simulink model "RLmodel"  (R2025b)
settings: Solver=FixedStepAuto  StartTime=0.0  StopTime=20.05  FixedStep=0.001  RelTol=1e-5  AbsTol=1e-6
model workspace (MAT data in the model file):
  I = 0
  c = 0
  g = 9.81
  l = 1
  m = 1
  max_tau = 2
undefined symbols (not defined in the file): x0
settings Model: Creator=The MathWorks, Inc.  LastModifiedBy=lengj
settings SolverCC: AutoScaleAbsTol=off  AlgebraicLoopSolver=TrustRegion
settings DataIOCC: LimitDataPoints=on  SaveFormat=Array  SaveState=on
settings OptimizationCC: BlockReduction=off  BooleanDataType=off  LifeSpan=inf
settings DebuggingCC: SaveWithParameterizedLinksMsg=none  SignalResolutionControl=TryResolveAllWithWarning  UnconnectedInputMsg=warning  UnconnectedOutputMsg=warning  UnconnectedLineMsg=warning  SFUnexpectedBacktrackingDiag=warning  SFNoUnconditionalDefaultTransitionDiag=warning  SFExecutionAtInitializationDiag=none  ArithmeticOperatorsInVariantConditions=warning
settings HardwareCC: ProdBitPerPointer=32.0  ProdBitPerSizeT=32.0  ProdBitPerPtrDiffT=32.0  ProdLargestAtomicFloat=None  ProdIntDivRoundTo=Undefined  ProdEndianess=Unspecified  ProdWordSize=32.0  ProdHWDeviceType=32-bit Generic  TargetUnknown=on
settings ModelReferenceCC: EnableRefExpFcnMdlSchedulingChecks=on  PropagateSignalLabelsOutOfModel=off
settings SFSimCC: SimUseLocalCustomCode=off  CustomCodeUndefinedFunction=UseInterfaceOnly
settings RTWCC: RTWUseLocalCustomCode=off  GPUComputeCapability=3.5
settings CodeAppCC: StateflowObjectComments=on
settings GRTTargetCC: TargetLangStandard=C89/C90 (ANSI)
settings ConfigComp: CovMetricSettings=dw  CovSaveCumulativeToWorkspaceVar=on  CovSaveSingleToWorkspaceVar=on  CovExternalEMLEnable=off

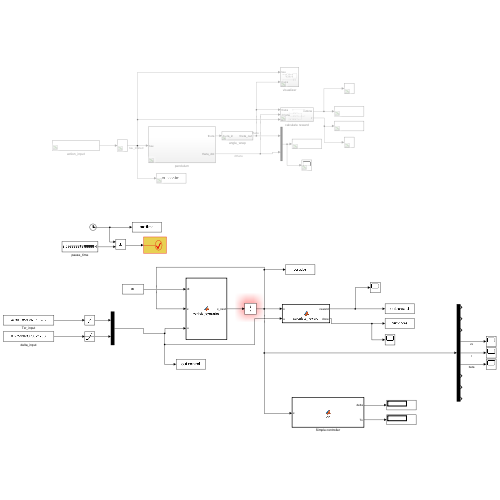
[thumbnail: Simulink's stored preview of the top-level diagram]
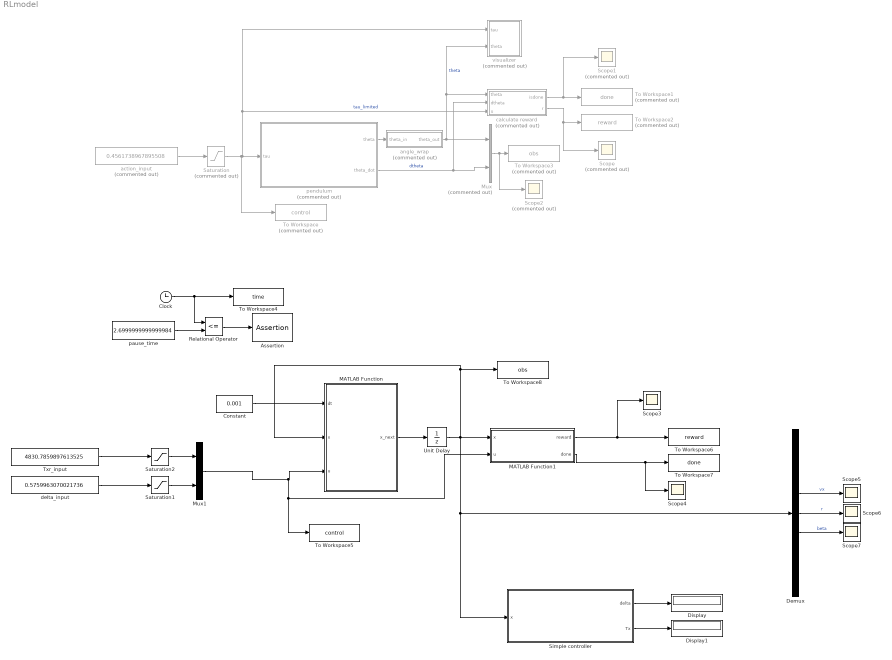
== system RLmodel ==
  Assertion : Assertion  AssertionFailFcn=set_param(bdroot,'SimulationCommand','pause')  StopWhenAssertionFail=off
  Clock : Clock
  Constant : Constant  Value=0.001
  Demux : Demux  Outputs=9
  Display : Display
  Display1 : Display
  MATLAB Function : MATLAB Function  TreatAsAtomicUnit=on
  MATLAB Function1 : MATLAB Function  TreatAsAtomicUnit=on
  Mux : Mux  Commented=on  Inputs=2
  Mux1 : Mux  Inputs=2
  Relational Operator : RelationalOperator  Operator=<=  OutDataTypeStr=boolean  RndMeth=Simplest  InputSameDT=off
  Saturation : Saturate  Commented=on  UpperLimit=max_tau  LowerLimit=-max_tau
  Saturation1 : Saturate  UpperLimit=35/180*pi  LowerLimit=-35/180*pi
  Saturation2 : Saturate  UpperLimit=5000  LowerLimit=-5000
  Scope : Scope  Commented=on
      settings: ActiveDisplayYMinimum=-25.392205164874287  ActiveDisplayYMaximum=34.906863641276743
  Scope1 : Scope  Commented=on
      settings: ActiveDisplayYMinimum=-1  ActiveDisplayYMaximum=1  DataLoggingVariableName=ScopeData2
  Scope2 : Scope  Commented=on
      settings: ActiveDisplayYMinimum=-1  ActiveDisplayYMaximum=1  DataLoggingVariableName=ScopeData3
  Scope{3..7} (5 alike) : Scope
      Scope3 settings: ActiveDisplayYMinimum=-9.323040755120104  ActiveDisplayYMaximum=43.32477207573163  DataLoggingVariableName=ScopeData4
      Scope4 settings: ActiveDisplayYMinimum=-1.1970312500000002  ActiveDisplayYMaximum=1.11821875  DataLoggingVariableName=ScopeData5
      Scope5 settings: ActiveDisplayYMinimum=-1  ActiveDisplayYMaximum=1  DataLoggingVariableName=ScopeData6
      Scope6 settings: ActiveDisplayYMinimum=-1  ActiveDisplayYMaximum=1  DataLoggingVariableName=ScopeData7
      Scope7 settings: ActiveDisplayYMinimum=-1  ActiveDisplayYMaximum=1  DataLoggingVariableName=ScopeData8
  Simple controller : MATLAB Function  TreatAsAtomicUnit=on
  To Workspace : ToWorkspace  Commented=on  VariableName=control  SaveFormat=Timeseries  SampleTime=-1
  To Workspace1 : ToWorkspace  Commented=on  VariableName=done  SaveFormat=Timeseries  SampleTime=-1
  To Workspace2 : ToWorkspace  Commented=on  VariableName=reward  SaveFormat=Timeseries  SampleTime=-1
  To Workspace3 : ToWorkspace  Commented=on  VariableName=obs  SaveFormat=Timeseries  SampleTime=-1
  To Workspace4 : ToWorkspace  VariableName=time  SaveFormat=Timeseries  SampleTime=-1
  To Workspace5 : ToWorkspace  VariableName=control  SaveFormat=Timeseries  SampleTime=-1
  To Workspace6 : ToWorkspace  VariableName=reward  SaveFormat=Timeseries  SampleTime=-1
  To Workspace7 : ToWorkspace  VariableName=done  SaveFormat=Timeseries  SampleTime=-1
  To Workspace8 : ToWorkspace  VariableName=obs  SaveFormat=Timeseries  SampleTime=-1
  Txr_input : Constant  Value=4830.7859897613525
  Unit Delay : UnitDelay  InitialCondition=x0  SampleTime=-1  HasFrameUpgradeWarning=on
  action_input : Constant  Commented=on  Value=0.4561738967895508
  angle_wrap : Subsystem  Commented=on
  calculate reward : Subsystem  Commented=on
  delta_input : Constant  Value=0.5759963070021736
  pause_time : Constant  Value=2.6999999999999984
  pendulum : Subsystem  Commented=on
  visualizer : Subsystem  Commented=on
  wires:
  Relational Operator/1 -> Assertion/1
  pendulum/2(theta_dot) -> calculate reward/2(dtheta), Mux/2  "dtheta"
  Clock/1 -> Relational Operator/1, To Workspace4/1
  angle_wrap/1(theta_out) -> Mux/1, visualizer/2(theta), calculate reward/1(theta)  "theta"
  calculate reward/1(isdone) -> Scope1/1, To Workspace1/1
  Saturation/1 -> To Workspace/1, visualizer/1(tau), calculate reward/3(u), pendulum/1(tau)  "tau_limited"
  pendulum/1(theta) -> angle_wrap/1(theta_in)
  action_input/1 -> Saturation/1
  pause_time/1 -> Relational Operator/2
  calculate reward/2(r) -> Scope/1, To Workspace2/1
  Mux/1 -> Scope2/1, To Workspace3/1
  Constant/1 -> MATLAB Function/1(dt)
  MATLAB Function/1(x_next) -> Unit Delay/1
  Unit Delay/1 -> Simple controller/1(x), Demux/1, MATLAB Function/2(x), To Workspace8/1, MATLAB Function1/1(x)
  Mux1/1 -> MATLAB Function1/2(u), To Workspace5/1, MATLAB Function/3(u)
  Saturation1/1 -> Mux1/2
  Saturation2/1 -> Mux1/1
  MATLAB Function1/1(reward) -> Scope3/1, To Workspace6/1
  MATLAB Function1/2(done) -> To Workspace7/1, Scope4/1
  Demux/4 -> Scope5/1  "vx"
  Demux/5 -> Scope6/1  "r"
  Demux/6 -> Scope7/1  "beta"
  Txr_input/1 -> Saturation2/1
  delta_input/1 -> Saturation1/1
  Simple controller/1(delta) -> Display/1
  Simple controller/2(Tx) -> Display1/1

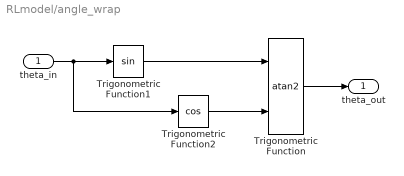
== system RLmodel/angle_wrap ==
  theta_in : Inport
  Trigonometric Function : Trigonometry  Operator=atan2
  Trigonometric Function1 : Trigonometry
  Trigonometric Function2 : Trigonometry  Operator=cos
  theta_out : Outport  VectorParamsAs1DForOutWhenUnconnected=off
  wires:
  theta_in/1 -> Trigonometric Function2/1, Trigonometric Function1/1
  Trigonometric Function/1 -> theta_out/1
  Trigonometric Function1/1 -> Trigonometric Function/1
  Trigonometric Function2/1 -> Trigonometric Function/2

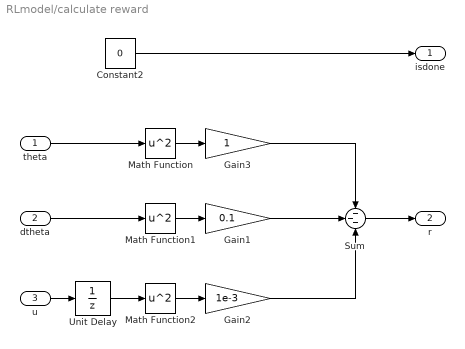
== system RLmodel/calculate reward ==
  theta : Inport
  dtheta : Inport  Port=2
  u : Inport  Port=3
  Constant2 : Constant  Value=0
  Gain1 : Gain  Gain=0.1
  Gain2 : Gain  Gain=1e-3
  Gain3 : Gain
  Math Function : Math  Operator=square  SignedPower=on
  Math Function1 : Math  Operator=square  SignedPower=on
  Math Function2 : Math  Operator=square  SignedPower=on
  Sum : Sum  Inputs=---
  Unit Delay : UnitDelay  SampleTime=-1  HasFrameUpgradeWarning=on
  isdone : Outport  VectorParamsAs1DForOutWhenUnconnected=off
  r : Outport  Port=2  VectorParamsAs1DForOutWhenUnconnected=off
  wires:
  Constant2/1 -> isdone/1
  theta/1 -> Math Function/1
  dtheta/1 -> Math Function1/1
  u/1 -> Unit Delay/1
  Sum/1 -> r/1
  Math Function/1 -> Gain3/1
  Math Function1/1 -> Gain1/1
  Math Function2/1 -> Gain2/1
  Gain2/1 -> Sum/3
  Gain1/1 -> Sum/2
  Gain3/1 -> Sum/1
  Unit Delay/1 -> Math Function2/1

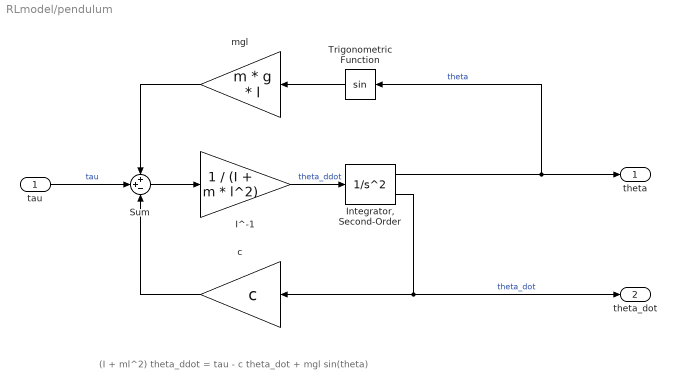
== system RLmodel/pendulum ==
  note: (I + ml^2) theta_ddot = tau - c theta_dot + mgl sin(theta)
  tau : Inport
  I^-1 : Gain  Gain=1 / (I + m * l^2)
  "Integrator, Second-Order" : SecondOrderIntegrator  ICX=theta0  UpperLimitX=1  LowerLimitX=0  StateNameX='theta'  ICDXDT=theta_dot0  StateNameDXDT='theta_dot'
  Sum : Sum  Inputs=++-
  Trigonometric Function : Trigonometry
  c : Gain  Gain=c
  mgl : Gain  Gain=m * g * l
  theta : Outport  VectorParamsAs1DForOutWhenUnconnected=off
  theta_dot : Outport  Port=2  VectorParamsAs1DForOutWhenUnconnected=off
  wires:
  mgl/1 -> Sum/1
  c/1 -> Sum/3
  Trigonometric Function/1 -> mgl/1
  Sum/1 -> I^-1/1
  "Integrator, Second-Order"/1 -> theta/1, Trigonometric Function/1  "theta"
  I^-1/1 -> "Integrator, Second-Order"/1  "theta_ddot"
  "Integrator, Second-Order"/2 -> c/1, theta_dot/1  "theta_dot"
  tau/1 -> Sum/2  "tau"

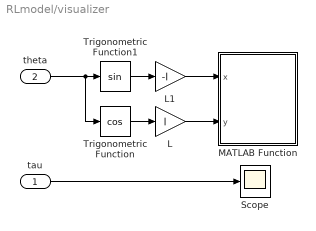
== system RLmodel/visualizer ==
  tau : Inport
  theta : Inport  Port=2
  L : Gain  Gain=l
  L1 : Gain  Gain=-l
  MATLAB Function : MATLAB Function  TreatAsAtomicUnit=on
  Scope : Scope
      settings: ActiveDisplayYMinimum=-2.2  ActiveDisplayYMaximum=2.2
  Trigonometric Function : Trigonometry  Operator=cos
  Trigonometric Function1 : Trigonometry
  wires:
  theta/1 -> Trigonometric Function/1, Trigonometric Function1/1
  L1/1 -> MATLAB Function/1(x)
  Trigonometric Function/1 -> L/1
  L/1 -> MATLAB Function/2(y)
  Trigonometric Function1/1 -> L1/1
  tau/1 -> Scope/1

== matlab function RLmodel/MATLAB Function ==
  data: dt input; x input; u input; x_next output
function x_next = vehicle_dynamics(dt, x, u)
% VEHICLE_DYNAMICS 3DOF车辆动力学模型 (Frenet坐标系)
% 目标：在直道上从任意初始状态恢复稳定并快速通行
% 
% 状态 x (6维): [s, e, mu, vx, r, beta]
% 动作 u (2维): [Fx_req, delta] (驱动力, 前轮转角)

% ==================== 1. 参数定义 ====================
% 物理参数
m = 1500;       % 质量 (kg)
Iz = 2250;      % 转动惯量 (kg·m^2)
lf = 1.2;       % 质心到前轴距离 (m)
lr = 1.6;       % 质心到后轴距离 (m)
L = lf + lr;    % 轴距
g = 9.81;
hcg = 0.5;
Rw = 0.353;
Jw = 0.9;

% 轮胎参数 (简化版 Magic Formula)
B = 15.2890; C = 1.0901; D = 0.60; E = 0.8621;
% D = mu_road * Fz，这里简化假设 D 为峰值摩擦系数 * 归一化载荷

% ==================== 2. 状态提取 ====================
s     = x(1);    % 纵向位置 (m)
e     = x(2);    % 侧向偏差 (m)
mu    = x(3);    % 航向角误差 (rad)
vx    = x(4);    % 纵向速度 (m/s)
r     = x(5);    % 横摆角速度 (rad/s)
beta  = x(6);    % 质心侧偏角 (rad)
ax    = x(7);
omega_r = x(8);
vy    = x(9);

% ==================== 3. 控制输入提取 ====================
Txr    = u(1);   % 纵向驱动/制动力 (N)
delta  = u(2);   % 前轮转角 (rad)

% ==================== 4. 中间变量计算 ====================
% 速度分量
v = vx / cos(beta);      % 侧向速度

% 轮胎侧偏角 (Slip Angles)
% 前轮侧偏角 alpha_f = atan((vy + lf*r)/vx) - delta
% 小角度假设下：
alpha_f = (vy + lf * r) / vx - delta; % 加max防止除零
alpha_r = (vy - lr * r) / vx;

% 垂直载荷 (静态分布)
Fzf = m / L * (g * lr - ax * hcg);
Fzr = m / L * (g * lf + ax * hcg);

% 纵向滑移率计算
lambda_r = (omega_r * Rw - vx) / vx;

% 后轮
sigma_x = lambda_r / (1 + lambda_r);
sigma_y = alpha_r / (1 + lambda_r);
sigma = sqrt(sigma_x * sigma_x + sigma_y * sigma_y);
% 后轮采用
FR = D * sin(C * atan(B * sigma - E * (B * sigma - atan(B * sigma)))) * Fzr;
FyR = - FR * sigma_y / sigma;
FxR = FR * sigma_x / sigma;

FyF = -D * sin(C * atan(B * alpha_f - E * (B * alpha_f - atan(B * alpha_f)))) * Fzf;

% 道路曲率 (直线赛道 k=0)
kappa = 0; 

% ==================== 5. 状态导数计算 ====================
% --- 运动学 (Frenet Frame) ---
% 分母项 den = 1 - e * kappa，直线时为 1
s_dot  = (v * cos(mu + beta)) / (1 - e * kappa);
e_dot  = v * sin(mu + beta);
mu_dot = r - kappa * s_dot;

% --- 动力学 (Newton-Euler) ---
% 1. 纵向加速度: m(vx_dot - r*vy) = Fx - FyF*sin(delta) - Drag
% 这里忽略风阻，或者你可以加回去
ax_next = 1 / m * (FxR - FyF * sin(delta));
vx_dot = ax_next + r * vy;

% 2. 侧向动力学 (用 beta_dot 表示): 
% m(vy_dot + r*vx) = FyF*cos(delta) + FyR
% beta_dot approx (FyF + FyR)/(m*vx) - r
vy_dot = 1 / m * (FyR + FyF * cos(delta)) - r * vx;

% 3. 横摆动力学: Iz * r_dot = lf*FyF*cos(delta) - lr*FyR
r_dot = (lf * FyF * cos(delta) - lr * FyR) / Iz;

omega_r_dot = (Txr - Rw * FxR) / Jw;

% ==================== 6. 积分 (欧拉法) ====================
s_next    = s + dt * s_dot;
e_next    = e + dt * e_dot;
mu_next   = mu + dt * mu_dot;
vx_next   = vx + dt * vx_dot;
vy_next   = vy + dt * vy_dot;
r_next    = r + dt * r_dot;
beta_next = atan(vy_next / vx_next);
omega_r_next = omega_r + dt * omega_r_dot;

x_next = [s_next, e_next, mu_next, vx_next, r_next, beta_next, ax_next, omega_r_next, vy_next];
end

== matlab function RLmodel/visualizer/MATLAB Function ==
  settings: updateMethod=DISCRETE
  data: x input; y input
function plotPend(x,y)
% plot the simple pendulum
coder.extrinsic('rl.env.viz.plotSimplePendulum');
rl.env.viz.plotSimplePendulum(x,y);

== matlab function RLmodel/MATLAB Function1 ==
  data: x input; reward output; u input; done output
function [reward, done] = calculate_reward(x, u)

s = x(1);
e = x(2);
mu = x(3);
vx = x(4);
r = x(5);
beta = x(6);

Fx = u(1);
delta = u(2);

% progress reward. 鼓励向前移动，速度越快奖励越高
reward_progress = 1.0 * (vx * cos(mu));

% stability penalty. 惩罚大侧偏角和横摆角速度
reward_stability = -2.0 * abs(mu) - 5.0 * abs(beta) - 0.5 * abs(r);

% Control effort. 避免方向盘高频抖动
reward_action = -0.1 * delta * delta;

% Terminal conditions
reward_terminal = 0;

% 冲出赛道
if abs(e) > 5.0
    reward_terminal = -1000.0;
    done = 1;
% 完成比赛
elseif s >= 200.0
    reward_terminal = 200.0;
    done = 2;
% 车辆失控
elseif abs(mu) > 2/3*pi
    reward_terminal = -1000.0;
    done = 3;
% 未完成
else
    done = -1;
end

reward = reward_progress + reward_stability + reward_action + reward_terminal;

== matlab function RLmodel/Simple controller ==
  data: x input; delta output; Tx output
function [delta, Tx] = fcn(x)

% ==================== 2. 状态提取 ====================
s     = x(1);    % 纵向位置 (m)
e     = x(2);    % 侧向偏差 (m)
mu    = x(3);    % 航向角误差 (rad)
vx    = x(4);    % 纵向速度 (m/s)
r     = x(5);    % 横摆角速度 (rad/s)
beta  = x(6);    % 质心侧偏角 (rad)
ax    = x(7);
omega_r = x(8);
vy    = x(9);

k_mu = 0.7;
k_r = 0.2;
k_beta = 0.2;

steer = -(k_mu * mu) - k_r * r - k_beta * beta;
steer = min(steer, 30/180*pi);
steer = max(steer, -30*180/pi);

if abs(beta) > 0.20 || abs(r) > 0.20
    throttle = 0;
elseif abs(beta) < 0.05 && abs(r) < 0.05
    throttle = 1.0;
else
    throttle = 6.7 * (abs(r) - 0.05);
end
Tx = throttle * 1000.0;
delta = steer;
